simulink model "ECE453_EXAM_FINAL"  (R2025a)
settings: Solver=VariableStepAuto  StartTime=0.0  StopTime=.05  RelTol=1e-3
model workspace (MAT data in the model file):
  Var = 0
settings Model: Creator=cruisemac  LastModifiedBy=cruisemac

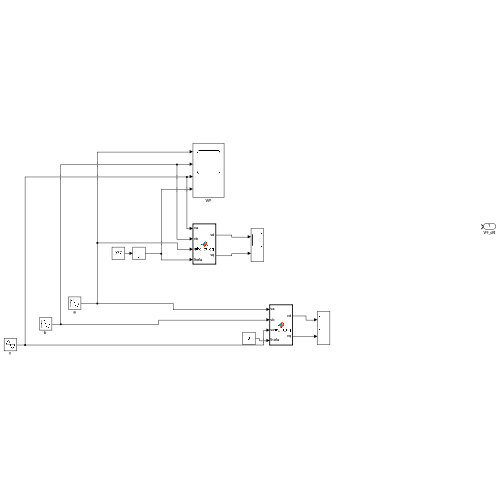
[thumbnail: Simulink's stored preview of the top-level diagram]
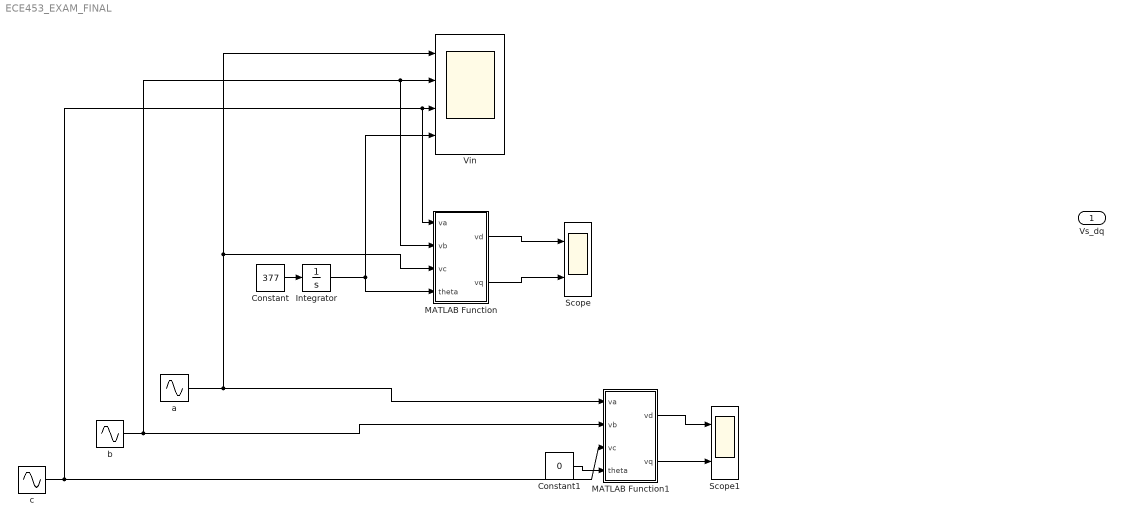
== system ECE453_EXAM_FINAL ==
  Constant : Constant  Value=377
  Constant1 : Constant  Value=0
  Integrator : Integrator
  MATLAB Function : MATLAB Function  TreatAsAtomicUnit=on
  MATLAB Function1 : MATLAB Function  TreatAsAtomicUnit=on
  Scope : Scope  NumInputPorts=2
      settings: ActiveDisplayYMinimum=-1  ActiveDisplayYMaximum=1
  Scope1 : Scope  NumInputPorts=2
      settings: ActiveDisplayYMinimum=-244.93699551158767  ActiveDisplayYMaximum=244.84116537774585
  Vin : Scope  NumInputPorts=4
      settings: ActiveDisplayYMinimum=-173.20488217112788  ActiveDisplayYMaximum=173.20456629580386  DataLoggingVariableName=ScopeData2
  a : Sin  Amplitude=240/sqrt(3) * sqrt(2)  Frequency=2*pi*60  SampleTime=0
  b : Sin  Amplitude=240/sqrt(3) * sqrt(2)  Frequency=2*pi*60  Phase=(-120/360)*2*pi  SampleTime=0
  c : Sin  Amplitude=240/sqrt(3) * sqrt(2)  Frequency=2*pi*60  Phase=(120/360)*2*pi  SampleTime=0
  Vs_dq : Outport
  wires:
  b/1 -> MATLAB Function1/2(vb), Vin/2, MATLAB Function/2(vb)
  c/1 -> MATLAB Function1/3(vc), MATLAB Function/1(va), Vin/3
  a/1 -> MATLAB Function1/1(va), MATLAB Function/3(vc), Vin/1
  Integrator/1 -> MATLAB Function/4(theta), Vin/4
  Constant/1 -> Integrator/1
  Constant1/1 -> MATLAB Function1/4(theta)
  MATLAB Function/2(vq) -> Scope/2
  MATLAB Function/1(vd) -> Scope/1
  MATLAB Function1/1(vd) -> Scope1/1
  MATLAB Function1/2(vq) -> Scope1/2

== matlab function ECE453_EXAM_FINAL/MATLAB Function1 ==
  data: va input; vd output; vb input; vc input; theta input; vq output
function [vd, vq] = abc_to_dq(va, vb,vc, theta)

vd = (2/3)*(va*cos(theta) ...
    + vb*cos(theta - 2*pi/3) ...
    + vc*cos(theta + 2*pi/3));

vq = -(2/3)*(va*sin(theta) ...
    + vb*sin(theta - 2*pi/3) ...
    + vc*sin(theta + 2*pi/3));

end

== matlab function ECE453_EXAM_FINAL/MATLAB Function ==
  data: va input; vd output; vb input; vc input; theta input; vq output
function [vd, vq] = abc_to_dq(va, vb,vc, theta)

vd = (2/3)*(va*cos(theta) ...
    + vb*cos(theta - 2*pi/3) ...
    + vc*cos(theta + 2*pi/3));

vq = -(2/3)*(va*sin(theta) ...
    + vb*sin(theta - 2*pi/3) ...
    + vc*sin(theta + 2*pi/3));

end
